simulink model "filter"  (R2020a)
settings: Solver=VariableStepAuto  StartTime=0.0  StopTime=10.0  MaxStep=0.001  RelTol=1e-3
settings Model: Creator=Admin  LastModifiedBy=Admin

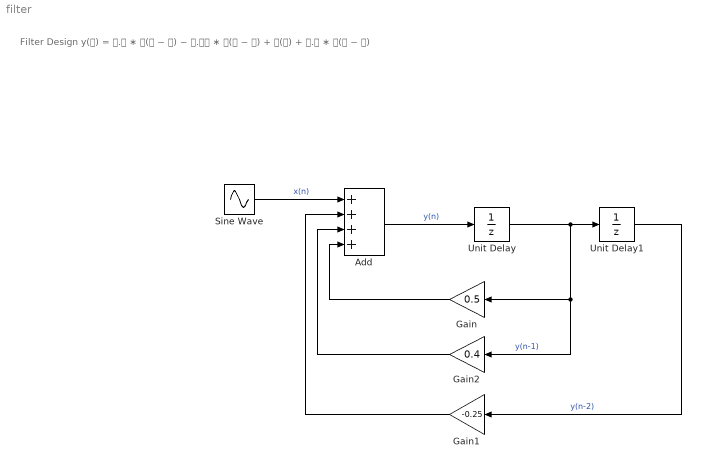
== system filter ==
  note: Filter Design
      | y(𝐧) = 𝟎.𝟓 ∗ 𝐲(𝐧 − 𝟏) − 𝟎.𝟐𝟓 ∗ 𝐲(𝐧 − 𝟐) + 𝐱(𝐧) + 𝟎.𝟒 ∗ 𝐱(𝐧 − 𝟏)
  Add : Sum  Inputs=++++
  Gain : Gain  Gain=0.5
  Gain1 : Gain  Gain=-0.25
  Gain2 : Gain  Gain=0.4
  Sine Wave : Sin  Frequency=10  SampleTime=0
  Unit Delay : UnitDelay  SampleTime=-1  HasFrameUpgradeWarning=on
  Unit Delay1 : UnitDelay  SampleTime=-1  HasFrameUpgradeWarning=on
  wires:
  Sine Wave/1 -> Add/1  "x(n)"
  Add/1 -> Unit Delay/1  "y(n)"
  Unit Delay/1 -> Gain/1, Gain2/1, Unit Delay1/1  "y(n-1)"
  Unit Delay1/1 -> Gain1/1  "y(n-2)"
  Gain/1 -> Add/4
  Gain1/1 -> Add/2
  Gain2/1 -> Add/3
